simulink model "task_7_model"  (R2023b)
settings: Solver=VariableStepAuto  StartTime=0.0  StopTime=10.0  RelTol=1e-3
values from neighbouring files (symbols this model uses):
  A = [0,mf*g*h/Jconst,0,-mf*g/Jconst; 1,0,0,0; 0,-g,0,0; 0,0,1,0]    [task_7.m]
  B = [1/Jconst;0;0;0]    [task_7.m]
  C = [0,0,0,1]    [task_7.m]
  k_obs = (alpha_obs(5)*eye(4) +alpha_obs(4)*A + alpha_obs(3)*A^2+           alpha_obs(2)*A^3 + alpha_obs(1)*A^4)*qT_obs    [task_7.m]
  kT_pi_d = kpi_d(1:4)-P*C    [task_7.m]
  P = 1/(C*inv(B*kT-A)*B)    [task_7.m]
  PI = -kpi(5)    [task_7.m]
  Ts = 125e-4    (= 0.0125)    [task_7.m]
settings Model: Creator=Krish  LastModifiedBy=Krish

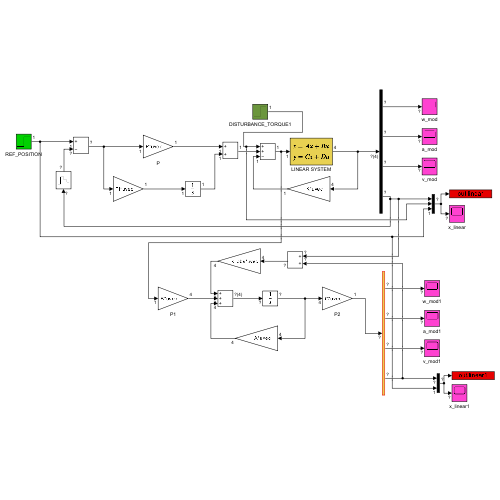
[thumbnail: Simulink's stored preview of the top-level diagram]
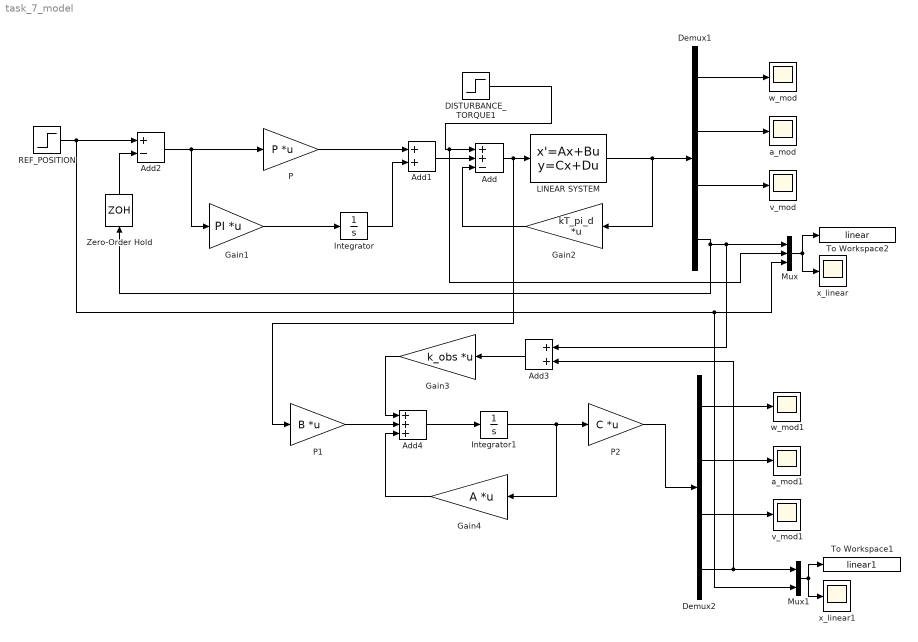
== system task_7_model ==
  Add : Sum  Inputs=++-
  Add1 : Sum
  Add2 : Sum  Inputs=+-
  Add3 : Sum
  Add4 : Sum  Inputs=+++
  DISTURBANCE_TORQUE1 : Step  Time=15  After=0.1  SampleTime=0
  Demux1 : Demux
  Demux2 : Demux
  Gain1 : Gain  Gain=PI  Multiplication=Matrix(K*u) (u vector)
  Gain2 : Gain  Gain=kT_pi_d  Multiplication=Matrix(K*u) (u vector)
  Gain3 : Gain  Gain=k_obs  Multiplication=Matrix(K*u) (u vector)
  Gain4 : Gain  Gain=A  Multiplication=Matrix(K*u) (u vector)
  Integrator : Integrator
  Integrator1 : Integrator
  LINEAR SYSTEM : StateSpace  A=A  B=B  C=eye(4)  D=[0;0;0;0]  InitialCondition=0
  Mux : Mux  Inputs=3
  Mux1 : Mux  Inputs=2
  P : Gain  Gain=P  Multiplication=Matrix(K*u) (u vector)
  P1 : Gain  Gain=B  Multiplication=Matrix(K*u) (u vector)
  P2 : Gain  Gain=C  Multiplication=Matrix(K*u) (u vector)
  REF_POSITION : Step  SampleTime=0
  To Workspace1 : ToWorkspace  VariableName=linear1  SaveFormat=Timeseries  SampleTime=-1
  To Workspace2 : ToWorkspace  VariableName=linear  SaveFormat=Timeseries  SampleTime=-1
  Zero-Order Hold : ZeroOrderHold  SampleTime=Ts
  a_mod : Scope
  a_mod1 : Scope
  v_mod : Scope
  v_mod1 : Scope
  w_mod : Scope
  w_mod1 : Scope
  x_linear : Scope
  x_linear1 : Scope
  wires:
  Add1/1 -> Add/2
  Mux/1 -> To Workspace2/1, x_linear/1
  Add/1 -> P1/1, LINEAR SYSTEM/1
  P/1 -> Add1/1
  DISTURBANCE_TORQUE1/1 -> Mux/2, Add/1
  Demux1/1 -> w_mod/1
  Zero-Order Hold/1 -> Add2/2
  Integrator/1 -> Add1/2
  Demux1/2 -> a_mod/1
  REF_POSITION/1 -> Add2/1, Mux1/2, Mux/3
  Gain1/1 -> Integrator/1
  Demux1/4 -> Zero-Order Hold/1, Mux/1, Add3/1
  Demux1/3 -> v_mod/1
  Gain2/1 -> Add/3
  LINEAR SYSTEM/1 -> Gain2/1, Demux1/1
  Add2/1 -> Gain1/1, P/1
  Add3/1 -> Gain3/1
  P1/1 -> Add4/2
  Add4/1 -> Integrator1/1
  Integrator1/1 -> Gain4/1, P2/1
  Gain4/1 -> Add4/3
  Gain3/1 -> Add4/1
  Demux2/1 -> w_mod1/1
  Demux2/2 -> a_mod1/1
  Demux2/3 -> v_mod1/1
  Demux2/4 -> Add3/2, Mux1/1
  Mux1/1 -> To Workspace1/1, x_linear1/1
  P2/1 -> Demux2/1
